simulink model "psbvoltmeasure"  (Simulink 6.0)
settings: Solver=ode15s  SolverMode=SingleTasking  StartTime=0.0  StopTime=0.1  RelTol=1e-3  AbsTol=1e-6
libraries: powerlib2 x14
settings Model: Creator=patrice  LastModifiedBy=batserve  ExtModeTrigMode=oneshot  ExtModeArmWhenConnect=off  ExtModeAutoUpdateStatusClock=off
settings DataIOCC: LimitDataPoints=off  SignalLoggingName=sigsOut
settings OptimizationCC: BooleanDataType=off
settings DebuggingCC: SolverPrmCheckMsg=none
settings HardwareCC: TargetUnknown=on
settings RTWCC: TemplateMakefile=grt_unix.tmf

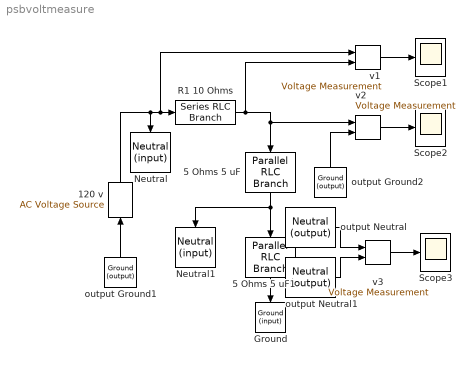
== system psbvoltmeasure ==
  120 v : powerlib2/Electrical Sources/AC Voltage Source  Tag=PoWeRsYsTeMbLoCk  Orientation=up  A=120  P=0  F=60  stime=0  mesure=None  PSBOutputType=1
  5 Ohms 5 uF : powerlib2/Elements/Parallel RLC Branch  Tag=PoWeRsYsTeMbLoCk  Orientation=down  a=5  b=inf  c=5e-06  mesure=None  PSBOutputType=1
  5 Ohms 5 uF1 : powerlib2/Elements/Parallel RLC Branch  Tag=PoWeRsYsTeMbLoCk  Orientation=down  a=3  b=inf  c=0  mesure=None  PSBOutputType=1
  Ground : powerlib2/Connectors/Ground (input)  Tag=PoWeRsYsTeMbLoCk  Orientation=down
  Neutral : powerlib2/Connectors/Neutral (input)  Tag=PoWeRsYsTeMbLoCk  Orientation=down  no=10
  Neutral1 : powerlib2/Connectors/Neutral (input)  Tag=PoWeRsYsTeMbLoCk  Orientation=down  no=20
  R1 10 Ohms : powerlib2/Elements/Series RLC Branch  Tag=PoWeRsYsTeMbLoCk  a=10  b=0  c=inf  mesure=None  PSBOutputType=1
  Scope1 : Scope
      settings: TickLabels=on  TimeRange=0.1  YMin=-100  YMax=100  DataFormat=Array
  Scope2 : Scope
      settings: TickLabels=on  TimeRange=0.1  YMin=-60  YMax=60  DataFormat=Array
  Scope3 : Scope
      settings: TickLabels=on  TimeRange=0.1  YMin=-120  YMax=120  DataFormat=Array
  output Ground1 : powerlib2/Connectors/Ground (output)  Tag=PoWeRsYsTeMbLoCk  Orientation=up  PSBOutputType=1
  output Ground2 : powerlib2/Connectors/Ground (output)  Tag=PoWeRsYsTeMbLoCk  Orientation=up  PSBOutputType=1
  output Neutral : powerlib2/Connectors/Neutral (output)  Tag=PoWeRsYsTeMbLoCk  no=10  PSBOutputType=1
  output Neutral1 : powerlib2/Connectors/Neutral (output)  Tag=PoWeRsYsTeMbLoCk  no=20  PSBOutputType=1
  v1 : powerlib2/Measurements/Voltage Measurement  Tag=PoWeRsYsTeMmEaSuReMeNt  PhasorSimulation=off  OutputType=Magnitude  PSBOutputType=0  PSBequivalent=0
  v2 : powerlib2/Measurements/Voltage Measurement  Tag=PoWeRsYsTeMmEaSuReMeNt  PhasorSimulation=off  OutputType=Magnitude  PSBOutputType=0  PSBequivalent=0
  v3 : powerlib2/Measurements/Voltage Measurement  Tag=PoWeRsYsTeMmEaSuReMeNt  PhasorSimulation=off  OutputType=Magnitude  PSBOutputType=0  PSBequivalent=0
  wires:
  output Neutral1/1 -> v3/2
  output Ground1/1 -> 120 v/1
  R1 10 Ohms/1 -> v1/2, 5 Ohms 5 uF/1, v2/1
  120 v/1 -> v1/1, R1 10 Ohms/1, Neutral/1
  5 Ohms 5 uF1/1 -> Ground/1
  5 Ohms 5 uF/1 -> Neutral1/1, 5 Ohms 5 uF1/1
  output Ground2/1 -> v2/2
  v2/1 -> Scope2/1
  v1/1 -> Scope1/1
  output Neutral/1 -> v3/1
  v3/1 -> Scope3/1
